simulink model "fuzzycontrollerPID"  (R2020b)
settings: Solver=VariableStepAuto  StartTime=0.0  StopTime=30  RelTol=1e-3
libraries: fuzblock x1
settings Model: Creator=Genesis Duque  LastModifiedBy=Genesis Duque

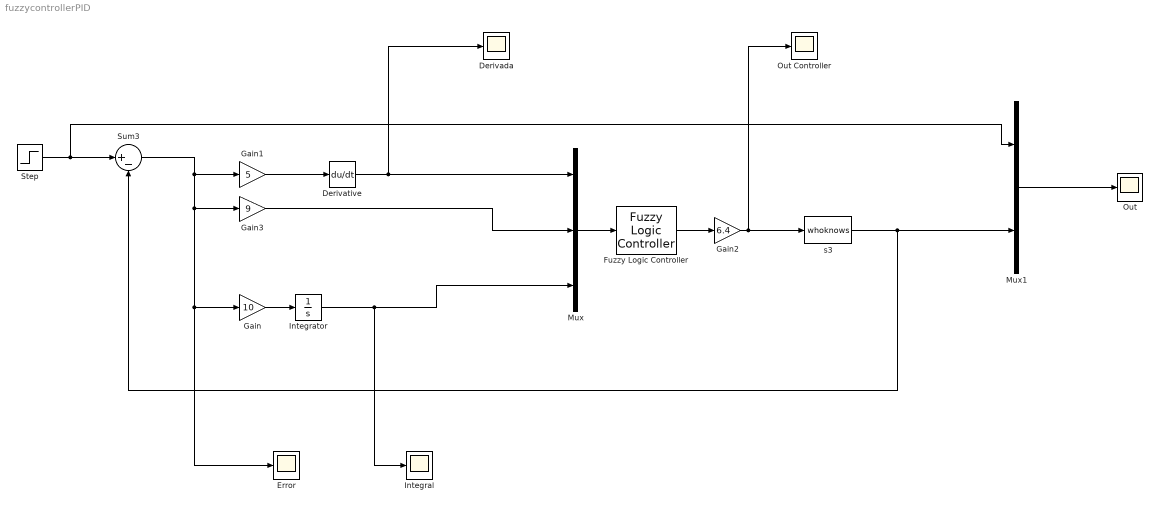
== system fuzzycontrollerPID ==
  Derivada : Scope
  Derivative : Derivative  CoefficientInTFapproximation=0.3209875
  Error : Scope
  Fuzzy Logic Controller : fuzblock/Fuzzy Logic  Controller  FIS='fuzzyPID.fis'  OutputSampleNumber=101  DataType=double  FuzzifiedInputs=off  RuleFiringStrengths=off  RuleOutputs=off  AggregatedOutputs=off  SimulateUsing=Interpreted execution  OutOfRangeInputValueMessage=warning  NoRuleFiredMessage=warning  EmptyOutputFuzzySetMessage=warning
  Gain : Gain  Gain=10
  Gain1 : Gain  Gain=5
  Gain2 : Gain  Gain=6.4
  Gain3 : Gain  Gain=9
  Integral : Scope
  Integrator : Integrator  InitialCondition=0.1692
  Mux : Mux  Inputs=3
  Mux1 : Mux  Inputs=2
  "Out " : Scope
  Out Controller : Scope
  Step : Step  SampleTime=0
  Sum3 : Sum  Inputs=|+-
  s3 : M-S-Function  FunctionName=whoknows  Parameters=L, P1, P2, T, R  mask{L=7, P1=0, P2=9, T=2, R=0}
      mask prompts: L "Laboratorio"; P1 "Primer digito del Puesto"; P2 "Segundo digito del Puesto"; T "Tipo de Planta"; R "Ruido"
      mask Display: disp('Sistema')
  wires:
  Step/1 -> Mux1/1, Sum3/1
  Mux1/1 -> "Out "/1
  Derivative/1 -> Derivada/1, Mux/1
  Sum3/1 -> Gain1/1, Gain3/1, Gain/1, Error/1
  Gain1/1 -> Derivative/1
  Gain3/1 -> Mux/2
  s3/1 -> Mux1/2, Sum3/2
  Gain2/1 -> Out Controller/1, s3/1
  Mux/1 -> Fuzzy Logic Controller/1
  Fuzzy Logic Controller/1 -> Gain2/1
  Integrator/1 -> Integral/1, Mux/3
  Gain/1 -> Integrator/1
